simulink model "ZZC_quadrotor_20251110"  (R2019b)
settings: Solver=ode4  StartTime=0.0  StopTime=20  FixedStep=1e-4
libraries: simulink x1
settings Model: Creator=bitgar  LastModifiedBy=zczhu

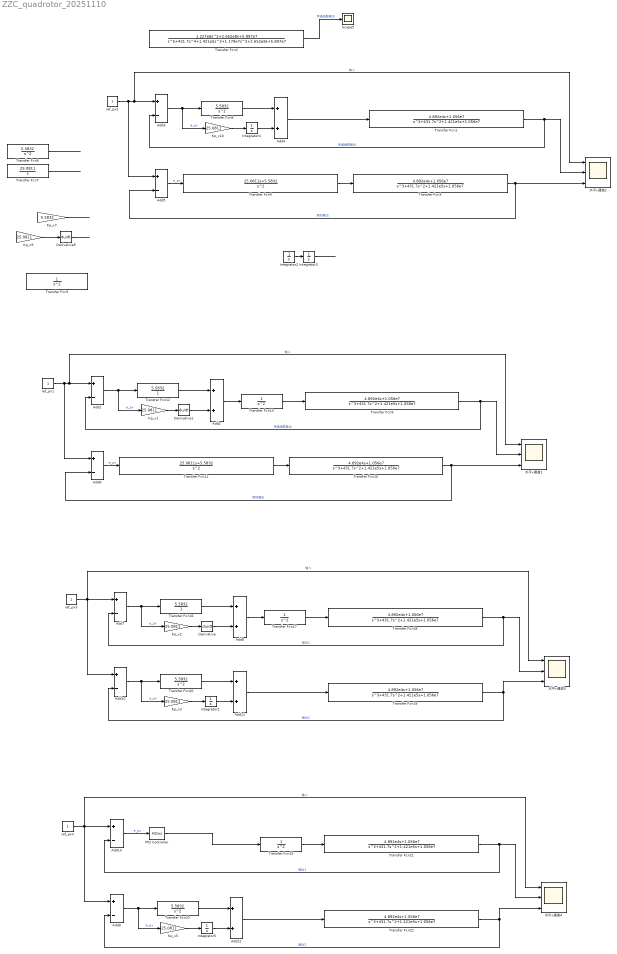
== system ZZC_quadrotor_20251110 ==
  Add{1,3,5..7,9..10,13} (8 alike) : Sum  Inputs=+-
  Add{2,4,8,11..12} (5 alike) : Sum
  Derivative : Derivative
  Derivative1 : Derivative
  Derivative5 : Derivative
  Integrator{1..5} (5 alike) : Integrator
  Kp_x{1..3,5,9..10} (6 alike) : Gain  Gain=25.0811
  Kp_x7 : Gain  Gain=5.5832
  PID Controller : simulink/Continuous/PID Controller  Controller=PID  Form=Parallel  TimeDomain=Continuous-time  SampleTime=-1  IntegratorMethod=Forward Euler  FilterMethod=Forward Euler  ControllerParametersSource=internal  P=5.5832  I=0  D=25.0811  UseFilter=on  N=1000  TunerSelectOption=Transfer Function Based (PID Tuner App)  InitialConditionSource=internal  InitialConditionForIntegrator=0  InitialConditionForFilter=0  DifferentiatorICPrevScaledInput=0  ExternalReset=none  TrackingMode=off  Kt=1  LimitOutput=off  UpperSaturationLimit=inf  LowerSaturationLimit=-inf  LinearizeAsGain=on  AntiWindupMode=none  Kb=1  POutMin=[]  POutMax=[]  IOutMin=[]  IOutMax=[]  DOutMin=[]  DOutMax=[]  NOutMin=[]  NOutMax=[]  SumOutMin=[]  SumOutMax=[]  SaturationOutMin=[]  SaturationOutMax=[]  PParamMin=[]  PParamMax=[]  IParamMin=[]  IParamMax=[]  DParamMin=[]  DParamMax=[]  NParamMin=[]  NParamMax=[]  KbParamMin=[]  KbParamMax=[]  KtParamMin=[]  KtParamMax=[]  KbOutMin=[]  KbOutMax=[]  KtOutMin=[]  KtOutMax=[]  IntegratorOutMin=[]  IntegratorOutMax=[]  FilterOutMin=[]  FilterOutMax=[]  SumI1OutMin=[]  SumI1OutMax=[]  SumI2OutMin=[]  SumI2OutMax=[]  SumI3OutMin=[]  SumI3OutMax=[]  SumI4OutMin=[]  SumI4OutMax=[]  SumDOutMin=[]  SumDOutMax=[]  DifferentiatorOutMin=[]  DifferentiatorOutMax=[]  FilterDiffOutCoefMin=[]  FilterDiffOutCoefMax=[]  ReciprocalOutMin=[]  ReciprocalOutMax=[]  SumDenOutMin=[]  SumDenOutMax=[]  SumNumOutMin=[]  SumNumOutMax=[]  DivideOutMin=[]  DivideOutMax=[]  IntegratorContinuousStateAttributes=''  IntegratorStateMustResolveToSignalObject=off  IntegratorRTWStateStorageClass=Auto  FilterContinuousStateAttributes=''  FilterStateMustResolveToSignalObject=off  FilterRTWStateStorageClass=Auto  ParallelPVariant=InternalParameters  IdealPVariant=Disabled  IVariant=InternalParameters  DVariant=InternalParameters  IntegratorVariant=Continuous  SatVariant=Disabled  AWVariant=Passthrough  PCopyVariant=Disabled  TRVariant=Disabled  FdbkBlocksVariant=Forward  IdealPFdbkVariant=Disabled  SatFdbkVariant=Disabled  DerivativeFilterVariant=ContFilter  NVariant=InternalParameters  NCopyVariant=Disabled  FilterICVariant=InternalICsFilter  IntegratorICVariant=InternalICs  ExternalResetVariant=Disabled  TRSumVariant=Passthrough  SumFdbkVariant=Disabled  SumVariant=Sum_PID
  Scope5 : Scope
  Transfer Fcn{1,3,9..10,18..19,21..22} (8 alike) : TransferFcn  Numerator=[4.892e4 1.056e7]  Denominator=[1 431.7 1.421e5 1.056e7]
  Transfer Fcn11 : TransferFcn  Numerator=[0 25.0811 5.5832]  Denominator=[1 0 0]
  Transfer Fcn12 : TransferFcn  Numerator=[5.5832]  Denominator=[1]
  Transfer Fcn{5,13,15,17} (4 alike) : TransferFcn  Denominator=[1 0 0]
  Transfer Fcn16 : TransferFcn  Numerator=[5.5832]  Denominator=[1]
  Transfer Fcn2 : TransferFcn  Numerator=[1.227e6 2.652e8 5.897e7]  Denominator=[1 431.7 1.421e5 1.179e7 2.652e8 5.897e7]
  Transfer Fcn{6,8,20,23} (4 alike) : TransferFcn  Numerator=[5.5832]  Denominator=[1 0 0]
  Transfer Fcn4 : TransferFcn  Numerator=[0 25.0811 5.5832]  Denominator=[1 0 0]
  Transfer Fcn7 : TransferFcn  Numerator=[25.0811]  Denominator=[1 0]
  ref_px{1..4} (4 alike) : Constant
  水平x通道{1..4} (4 alike) : Scope  NumInputPorts=3
  wires:
  Transfer Fcn2/1 -> Scope5/1  "传递函数输出"
  ref_px2/1 -> Add5/1, 水平x通道2/1, Add3/1  "输入"
  Add4/1 -> Transfer Fcn1/1
  Transfer Fcn1/1 -> 水平x通道2/2, Add3/2  "传递函数输出"
  Transfer Fcn4/1 -> Transfer Fcn3/1
  Add5/1 -> Transfer Fcn4/1  "e_px"
  Transfer Fcn3/1 -> Add5/2, 水平x通道2/3  "新的输出"
  Integrator3/1 -> ?
  Integrator2/1 -> Integrator3/1
  ? -> Kp_x9/1, Kp_x7/1  "e_px"
  Kp_x9/1 -> Derivative5/1
  Kp_x7/1 -> ?
  Derivative5/1 -> ?
  Add3/1 -> Kp_x10/1, Transfer Fcn8/1  "e_px"
  Transfer Fcn7/1 -> ?
  Transfer Fcn6/1 -> ?
  Transfer Fcn8/1 -> Add4/1
  Integrator4/1 -> Add4/2
  Kp_x10/1 -> Integrator4/1
  Transfer Fcn12/1 -> Add2/1
  Add1/1 -> Kp_x1/1, Transfer Fcn12/1  "e_px"
  Add6/1 -> Transfer Fcn11/1  "e_px"
  Kp_x1/1 -> Derivative1/1
  Transfer Fcn10/1 -> Add6/2, 水平x通道1/3  "新的输出"
  Add2/1 -> Transfer Fcn13/1
  ref_px1/1 -> Add6/1, 水平x通道1/1, Add1/1  "输入"
  Transfer Fcn11/1 -> Transfer Fcn10/1
  Transfer Fcn9/1 -> 水平x通道1/2, Add1/2  "传递函数输出"
  Transfer Fcn13/1 -> Transfer Fcn9/1
  Derivative1/1 -> Add2/2
  Transfer Fcn17/1 -> Transfer Fcn18/1
  Transfer Fcn18/1 -> 水平x通道3/2, Add7/2  "输出1"
  Derivative/1 -> Add8/2
  Add8/1 -> Transfer Fcn17/1
  Transfer Fcn16/1 -> Add8/1
  Kp_x2/1 -> Derivative/1
  Add7/1 -> Kp_x2/1, Transfer Fcn16/1  "e_px"
  Transfer Fcn20/1 -> Add11/1
  Integrator1/1 -> Add11/2
  Add10/1 -> Kp_x3/1, Transfer Fcn20/1  "e_px"
  Kp_x3/1 -> Integrator1/1
  ref_px3/1 -> 水平x通道3/1, Add7/1, Add10/1  "输入"
  Transfer Fcn19/1 -> 水平x通道3/3, Add10/2  "输出2"
  Add11/1 -> Transfer Fcn19/1
  Add13/1 -> PID Controller/1  "e_px"
  Add12/1 -> Transfer Fcn22/1
  Kp_x5/1 -> Integrator5/1
  Transfer Fcn22/1 -> 水平x通道4/3, Add9/2  "输出2"
  Transfer Fcn21/1 -> 水平x通道4/2, Add13/2  "输出1"
  Integrator5/1 -> Add12/2
  Add9/1 -> Kp_x5/1, Transfer Fcn23/1  "e_px"
  Transfer Fcn15/1 -> Transfer Fcn21/1
  ref_px4/1 -> 水平x通道4/1, Add13/1, Add9/1  "输入"
  Transfer Fcn23/1 -> Add12/1
  PID Controller/1 -> Transfer Fcn15/1
